simulink model "bebop_full"  (R2019b)
settings: Solver=VariableStepAuto  StartTime=0.0  StopTime=10.0  RelTol=1e-3
values from neighbouring files (symbols this model uses):
  Body_pos_damper = [ld; bd; 0] .* [1, -1, -1, 1;                                   1, 1, -1, -1;                                   0,0,0,0]    [MatToSimulink_test_tutorial.m]
  Damping_matrix_damper = eye(3) .* 1    [MatToSimulink_test_tutorial.m]
  delta_l0_body_frame = [ld; bd; delta_h_damper] .* [1,-1,-1, 1;                                                    1, 1,-1,-1 ... (first row only)    [MatToSimulink_test_tutorial.m]
  Elastic_matrix_damper = eye(3) .* 100    [MatToSimulink_test_tutorial.m]
  g = 9.81    [MatToSimulink_test_tutorial.m]
  Ib = diag([Ixxb, Iyyb, Izzb])    [MatToSimulink_test_tutorial.m]
  iIb = Ib \ eye(3)    [MatToSimulink_test_tutorial.m]
  k_t = 0.01    [MatToSimulink_test_tutorial.m]
  M_c = [b*k_t; l*k_t; k_tau] .* [-1 1 1 -1; 1 1 -1 -1; 1 -1 1 -1]    [MatToSimulink_test_tutorial.m]
  mb = 0.3    [MatToSimulink_test_tutorial.m]
  mc = 0.2    [MatToSimulink_test_tutorial.m]
  omega_c_propeller = 50    [MatToSimulink_test_tutorial.m]
libraries: vrlib x2
settings Model: Creator=ASUS  LastModifiedBy=ASUS

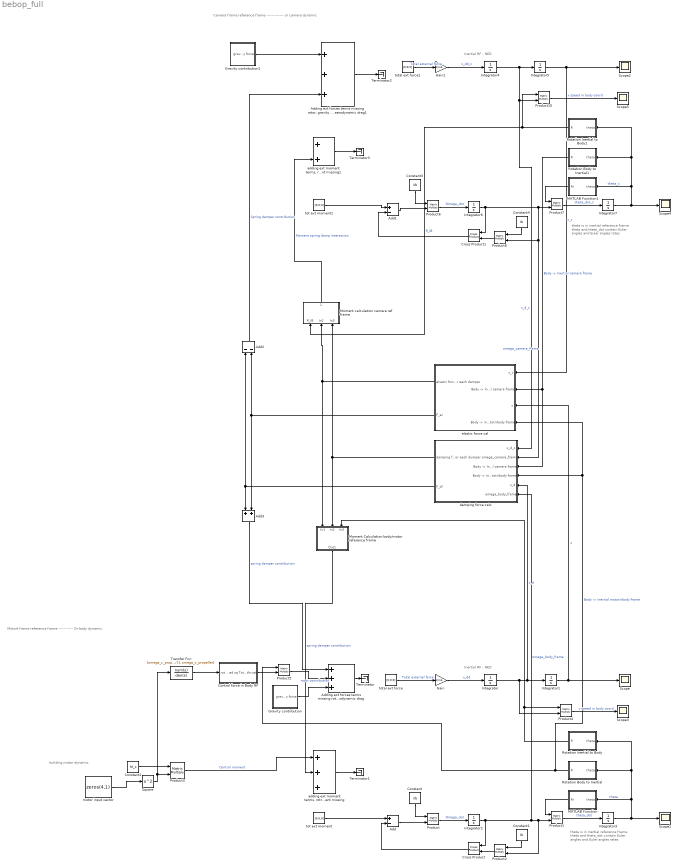
== system bebop_full ==
  note: Motort frame reference frame ----------- Or body dynamic
  note: building motor dynamic
  note: Inertial RF - NED
  note: theta is in inertial
      | reference frame
      |
      | theta and theta_dot contain
      | Euler angles and Euler angles rates
  note: Inertial RF - NED
  note: Camera frame reference frame ------------- or camera dynamic
  note: theta is in inertial
      | reference frame
      |
      | theta and theta_dot contain
      | Euler angles and Euler angles rates
  Add : Sum  Inputs=+-
  Add1 : Sum  Inputs=+-
  Add2 : Sum  Inputs=--
  Add3 : Sum
  "Adding ext forces terms missing rotor, gravity --Inertial Reference frame-- missing aerodynamic drag" : Sum  Inputs=+++
  "Adding ext forces terms missing rotor, gravity --Inertial Reference frame-- missing aerodynamic drag1" : Sum  Inputs=+++
  Constant : Constant  Value=iIb
  Constant1 : Constant  Value=Ib
  Constant2 : Constant  Value=M_c
  Constant3 : Constant  Value=iIb
  Constant4 : Constant  Value=Ib
  Control force in Body RF : Subsystem
  Cross Product : vrlib/Utilities/Cross Product
      settings: SourceProductName=Simulink
  Cross Product1 : vrlib/Utilities/Cross Product
      settings: SourceProductName=Simulink
  Gain : Gain  Gain=1/mb
  Gain1 : Gain  Gain=1/mb
  Gravity contribution : Subsystem
  Gravity contribution1 : Subsystem
  Integrator{,1..7} (8 alike) : Integrator  InitialCondition=[0;0;0]
  MATLAB Function : MATLAB Function  TreatAsAtomicUnit=on
  MATLAB Function1 : MATLAB Function  TreatAsAtomicUnit=on
  Moment Calculation body/motor reference frame : Subsystem
  Moment calculation camera ref frame : Subsystem
  Product{,1..8,10} (10 alike) : Product  Multiplication=Matrix(*)
  Rotation Body to Inertial : MATLAB Function  TreatAsAtomicUnit=on
  Rotation Body to Inertial1 : MATLAB Function  TreatAsAtomicUnit=on
  Rotation Inertial to Body : MATLAB Function  TreatAsAtomicUnit=on
  Rotation Inertial to Body1 : MATLAB Function  TreatAsAtomicUnit=on
  Scope{,1..5} (6 alike) : Scope
  Square : Math  Operator=square  SignedPower=off  SaturateOnIntegerOverflow=on
  Terminator{,1..3} (4 alike) : Terminator
  Transfer Fcn : TransferFcn  Numerator=[omega_c_propeller]  Denominator=[1 omega_c_propeller]
  "adding ext moment terms, rotr precession and aerodynamic moment missing" : Sum  Inputs=+++
  "adding ext moment terms, rotr precession and aerodynamic moment missing1" : Sum
  damping force calc : Subsystem
  elastic force cal : Subsystem
  "motor input vector " : Constant  Value=zeros(4,1)
  tot ext moment : Constant  Value=[0;0;0]
  tot ext moment1 : Constant  Value=[0;0;0]
  total ext force : Constant  Value=[0;0;0]
  total ext force1 : Constant  Value=[0;0;0]
  wires:
  Integrator/1 -> damping force calc/5(x_d), Integrator1/1, Product4/2  "x_d"
  Gain/1 -> Integrator/1  "x_dd"
  Integrator1/1 -> Scope/1, elastic force cal/3(x)  "x"
  total ext force/1 -> Gain/1  "Total external force"
  Product/1 -> Integrator2/1  "Omega_dot"
  tot ext moment/1 -> Add/1
  Constant/1 -> Product/1
  Add/1 -> Product/2
  Integrator2/1 -> Cross Product/1, damping force calc/6(omega_body_frame), Product2/2, Product1/2  "omega_body_frame"
  Integrator3/1 -> Rotation Inertial to Body/1(theta), Rotation Body to Inertial/1(theta), MATLAB Function/1(theta), Scope1/1  "theta"
  Product1/1 -> Integrator3/1  "theta_dot"
  MATLAB Function/1(Rr) -> Product1/1
  Product2/1 -> Cross Product/2
  Cross Product/1 -> Add/2
  Constant1/1 -> Product2/1
  Rotation Inertial to Body/1(R) -> Moment Calculation body/motor reference frame/3(In3), Product4/1
  Product4/1 -> Scope3/1  "v speed in body coord"
  Rotation Body to Inertial/1(R) -> elastic force cal/4("Body -> inertial mototr/body frame"), damping force calc/4("Body -> inertial mototr/body frame"), Product5/1  "Body -> inertial mototr/body frame"
  "motor input vector "/1 -> Square/1
  Constant2/1 -> Product3/1
  Product3/1 -> "adding ext moment terms, rotr precession and aerodynamic moment missing"/1  "Control moment"
  "adding ext moment terms, rotr precession and aerodynamic moment missing"/1 -> Terminator1/1
  Square/1 -> Transfer Fcn/1, Product3/2
  Product5/1 -> "Adding ext forces terms missing rotor, gravity --Inertial Reference frame-- missing aerodynamic drag"/2  "rotot contribution"
  Gravity contribution/1("gravity force ") -> "Adding ext forces terms missing rotor, gravity --Inertial Reference frame-- missing aerodynamic drag"/3
  "Adding ext forces terms missing rotor, gravity --Inertial Reference frame-- missing aerodynamic drag"/1 -> Terminator/1
  Control force in Body RF/1(Total thrust) -> Product5/2
  Add1/1 -> Product6/2
  Cross Product1/1 -> Add1/2
  "adding ext moment terms, rotr precession and aerodynamic moment missing1"/1 -> Terminator3/1
  Constant3/1 -> Product6/1
  Product7/1 -> Integrator7/1  "theta_dot_c"
  Rotation Inertial to Body1/1(R) -> Moment calculation camera ref frame/1(R_IB), Product10/1  "R_IB"
  Gravity contribution1/1("gravity force ") -> "Adding ext forces terms missing rotor, gravity --Inertial Reference frame-- missing aerodynamic drag1"/1
  Product8/1 -> Cross Product1/2
  MATLAB Function1/1(Rr) -> Product7/1
  tot ext moment1/1 -> Add1/1
  Product10/1 -> Scope5/1  "v speed in body coord"
  Integrator5/1 -> elastic force cal/1(x_c), Scope2/1  "x_c"
  Integrator6/1 -> Cross Product1/1, damping force calc/2(omega_camera_frame), Product8/2, Product7/2  "omega_camera_frame"
  Integrator7/1 -> Rotation Inertial to Body1/1(theta), Rotation Body to Inertial1/1(theta), MATLAB Function1/1(theta), Scope4/1  "theta_c"
  total ext force1/1 -> Gain1/1  "Total external force"
  Constant4/1 -> Product8/1
  Product6/1 -> Integrator6/1  "Omega_dot"
  "Adding ext forces terms missing rotor, gravity --Inertial Reference frame-- missing aerodynamic drag1"/1 -> Terminator2/1
  Gain1/1 -> Integrator4/1  "x_dd_c"
  Integrator4/1 -> damping force calc/1(x_d_c), Product10/2, Integrator5/1  "x_d_c"
  Rotation Body to Inertial1/1(R) -> damping force calc/3("Body -> Inertial camera frame"), elastic force cal/2("Body -> Inertial camera frame")  "Body -> Inertial camera frame"
  elastic force cal/1(elsatic force components for each damper) -> Moment calculation camera ref frame/2(In2), Moment Calculation body/motor reference frame/1(In1)
  elastic force cal/2(F_eI) -> Add2/2, Add3/2
  damping force calc/1(damping force components for each dumper) -> Moment Calculation body/motor reference frame/2(In2), Moment calculation camera ref frame/3(In3)
  damping force calc/2(F_dI) -> Add3/1, Add2/1
  Add2/1 -> "Adding ext forces terms missing rotor, gravity --Inertial Reference frame-- missing aerodynamic drag1"/3  "Spring damper contribution"
  Add3/1 -> "Adding ext forces terms missing rotor, gravity --Inertial Reference frame-- missing aerodynamic drag"/1  "spring damper contribution"
  Moment calculation camera ref frame/1(Spring-damper moment contribution) -> "adding ext moment terms, rotr precession and aerodynamic moment missing1"/2  "Moment spring damp interaction"
  Moment Calculation body/motor reference frame/1(Out1) -> "adding ext moment terms, rotr precession and aerodynamic moment missing"/2  "spring damper contribution"
  Transfer Fcn/1 -> Control force in Body RF/1(rot speed sq)

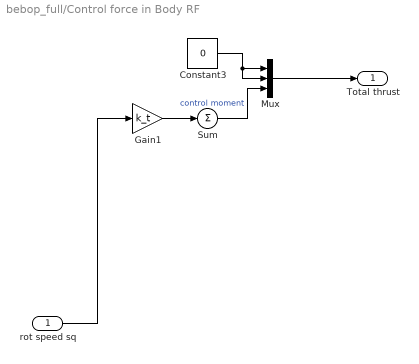
== system bebop_full/Control force in Body RF ==
  rot speed sq : Inport
  Constant3 : Constant  Value=0
  Gain1 : Gain  Gain=k_t
  Mux : Mux  Inputs=3
  Sum : Sum  Inputs=+
  Total thrust : Outport
  wires:
  Sum/1 -> Mux/3  "control moment"
  Constant3/1 -> Mux/1, Mux/2
  Mux/1 -> Total thrust/1
  Gain1/1 -> Sum/1
  rot speed sq/1 -> Gain1/1

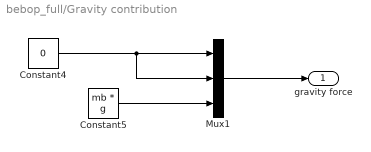
== system bebop_full/Gravity contribution ==
  Constant4 : Constant  Value=0
  Constant5 : Constant  Value=mb * g
  Mux1 : Mux  Inputs=3
  "gravity force " : Outport
  wires:
  Constant4/1 -> Mux1/1, Mux1/2
  Constant5/1 -> Mux1/3
  Mux1/1 -> "gravity force "/1

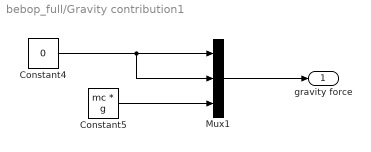
== system bebop_full/Gravity contribution1 ==
  Constant4 : Constant  Value=0
  Constant5 : Constant  Value=mc * g
  Mux1 : Mux  Inputs=3
  "gravity force " : Outport
  wires:
  Constant4/1 -> Mux1/1, Mux1/2
  Constant5/1 -> Mux1/3
  Mux1/1 -> "gravity force "/1

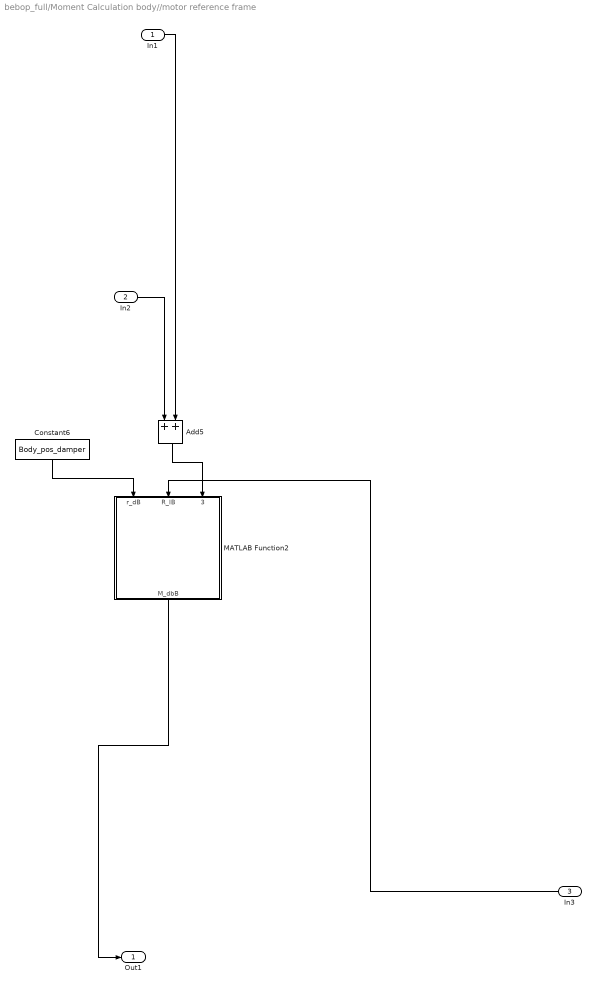
== system bebop_full/Moment Calculation body//motor reference frame ==
  In1 : Inport
  In2 : Inport  Port=2
  In3 : Inport  Port=3
  Add5 : Sum
  Constant6 : Constant  Value=Body_pos_damper
  MATLAB Function2 : MATLAB Function  TreatAsAtomicUnit=on
  Out1 : Outport
  wires:
  Add5/1 -> MATLAB Function2/3(F_dbI_comp)
  In1/1 -> Add5/2
  In2/1 -> Add5/1
  In3/1 -> MATLAB Function2/2(R_IB)
  Constant6/1 -> MATLAB Function2/1(r_dB)
  MATLAB Function2/1(M_dbB) -> Out1/1

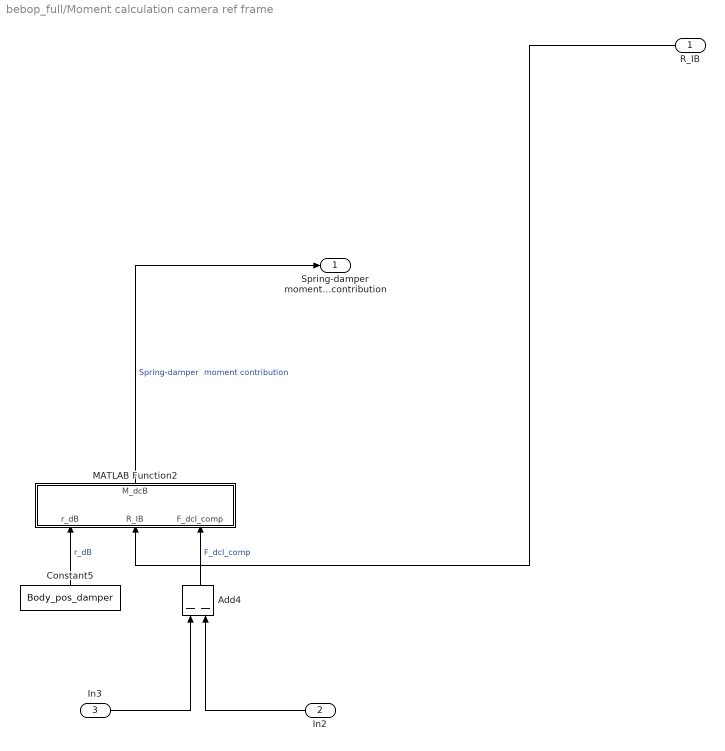
== system bebop_full/Moment calculation camera ref frame ==
  R_IB : Inport
  In2 : Inport  Port=2
  In3 : Inport  Port=3
  Add4 : Sum  Inputs=--
  Constant5 : Constant  Value=Body_pos_damper
  MATLAB Function2 : MATLAB Function  TreatAsAtomicUnit=on
  Spring-damper moment contribution : Outport
  wires:
  Add4/1 -> MATLAB Function2/3(F_dcI_comp)  "F_dcI_comp"
  MATLAB Function2/1(M_dcB) -> Spring-damper moment contribution/1  "Spring-damper  moment contribution"
  In3/1 -> Add4/1
  Constant5/1 -> MATLAB Function2/1(r_dB)  "r_dB"
  R_IB/1 -> MATLAB Function2/2(R_IB)
  In2/1 -> Add4/2

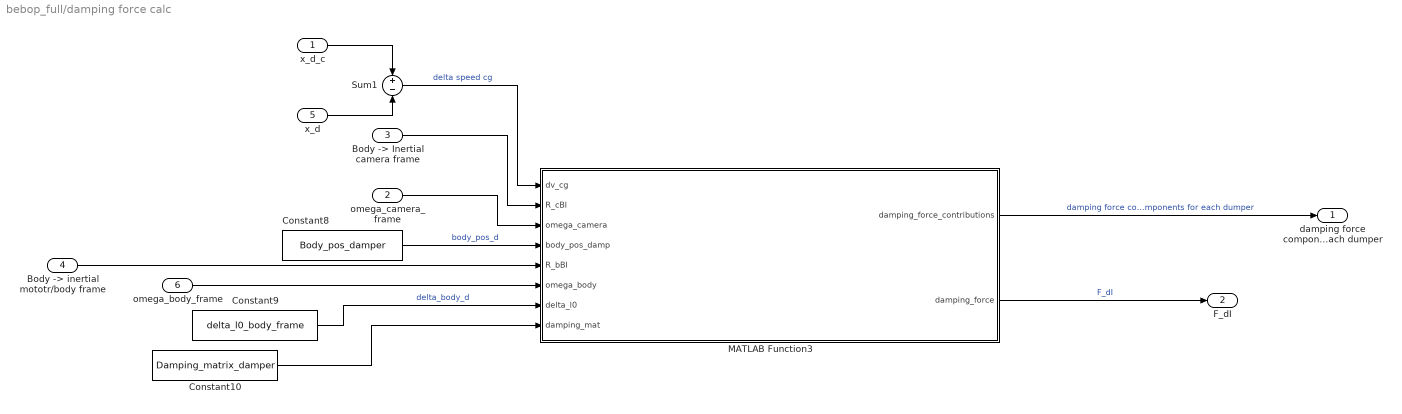
== system bebop_full/damping force calc ==
  x_d_c : Inport
  omega_camera_frame : Inport  Port=2
  "Body -> Inertial camera frame" : Inport  Port=3
  "Body -> inertial mototr/body frame" : Inport  Port=4
  x_d : Inport  Port=5
  omega_body_frame : Inport  Port=6
  Constant10 : Constant  Value=Damping_matrix_damper
  Constant8 : Constant  Value=Body_pos_damper
  Constant9 : Constant  Value=delta_l0_body_frame
  MATLAB Function3 : MATLAB Function  TreatAsAtomicUnit=on
  Sum1 : Sum  Inputs=+-
  damping force components for each dumper : Outport
  F_dI : Outport  Port=2
  wires:
  MATLAB Function3/2(damping_force) -> F_dI/1  "F_dI"
  x_d/1 -> Sum1/2
  x_d_c/1 -> Sum1/1
  "Body -> inertial mototr/body frame"/1 -> MATLAB Function3/5(R_bBI)
  omega_body_frame/1 -> MATLAB Function3/6(omega_body)
  omega_camera_frame/1 -> MATLAB Function3/3(omega_camera)
  Constant8/1 -> MATLAB Function3/4(body_pos_damp)  "body_pos_d"
  MATLAB Function3/1(damping_force_contributions) -> damping force components for each dumper/1  "damping force components for each dumper"
  Sum1/1 -> MATLAB Function3/1(dv_cg)  "delta speed cg"
  Constant10/1 -> MATLAB Function3/8(damping_mat)
  "Body -> Inertial camera frame"/1 -> MATLAB Function3/2(R_cBI)
  Constant9/1 -> MATLAB Function3/7(delta_l0)  "delta_body_d"

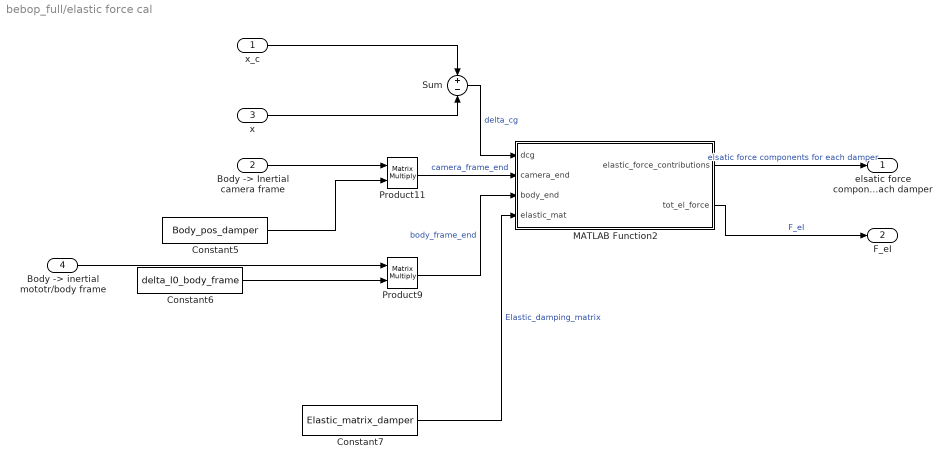
== system bebop_full/elastic force cal ==
  x_c : Inport
  "Body -> Inertial camera frame" : Inport  Port=2
  x : Inport  Port=3
  "Body -> inertial mototr/body frame" : Inport  Port=4
  Constant5 : Constant  Value=Body_pos_damper
  Constant6 : Constant  Value=delta_l0_body_frame
  Constant7 : Constant  Value=Elastic_matrix_damper
  MATLAB Function2 : MATLAB Function  TreatAsAtomicUnit=on
  Product11 : Product  Multiplication=Matrix(*)
  Product9 : Product  Multiplication=Matrix(*)
  Sum : Sum  Inputs=+-
  elsatic force components for each damper : Outport
  F_eI : Outport  Port=2
  wires:
  Constant6/1 -> Product9/2
  MATLAB Function2/2(tot_el_force) -> F_eI/1  "F_eI"
  "Body -> inertial mototr/body frame"/1 -> Product9/1
  Constant7/1 -> MATLAB Function2/4(elastic_mat)  "Elastic_damping_matrix"
  x_c/1 -> Sum/1
  x/1 -> Sum/2
  MATLAB Function2/1(elastic_force_contributions) -> elsatic force components for each damper/1  "elsatic force components for each damper"
  Product9/1 -> MATLAB Function2/3(body_end)  "body_frame_end"
  Product11/1 -> MATLAB Function2/2(camera_end)  "camera_frame_end"
  Constant5/1 -> Product11/2
  "Body -> Inertial camera frame"/1 -> Product11/1
  Sum/1 -> MATLAB Function2/1(dcg)  "delta_cg"

== matlab function bebop_full/Rotation Inertial to Body ==
  data: theta input; R output
function R = R_ItB(theta)

sp = sin(theta(1));
cp = cos(theta(1));

st = sin(theta(2));
ct = cos(theta(2));

ss = sin(theta(3));
cs = cos(theta(3));

R_Itv1 = [cs, ss, 0;...
          -ss, cs, 0;...
          0, 0, 1];

R_v1tv2 = [ct, 0, -st;...
           0, 1, 0;
           st, 0, ct];
       
R_v2tB = [1, 0, 0;...
          0, cp, sp;...
          0, -sp, cp];
      
R = R_v2tB * R_v1tv2 * R_Itv1;

== matlab function bebop_full/MATLAB Function ==
  data: theta input; Rr output
function Rr = rates_rot_mat(theta)

Rr = [1, sin(theta(1)).*tan(theta(2)), cos(theta(1)).*tan(theta(2));...
      0, cos(theta(1)), -sin(theta(1));...
      0, sin(theta(1))./cos(theta(2)), cos(theta(1))./cos(theta(2)) ];

== matlab function bebop_full/Rotation Body to Inertial ==
  data: theta input; R output
function R = R_BtI(theta)

sp = sin(-theta(1));
cp = cos(-theta(1));

st = sin(-theta(2));
ct = cos(-theta(2));

ss = sin(-theta(3));
cs = cos(-theta(3));

R_Itv1 = [cs, ss, 0;...
          -ss, cs, 0;...
          0, 0, 1];

R_v1tv2 = [ct, 0, -st;...
           0, 1, 0;
           st, 0, ct];
       
R_v2tB = [1, 0, 0;...
          0, cp, sp;...
          0, -sp, cp];
      
R =  R_Itv1 * R_v1tv2 * R_v2tB;

== matlab function bebop_full/MATLAB Function1 ==
  data: theta input; Rr output
function Rr = rates_rot_mat(theta)

Rr = [1, sin(theta(1)).*tan(theta(2)), cos(theta(1)).*tan(theta(2));...
      0, cos(theta(1)), -sin(theta(1));...
      0, sin(theta(1))./cos(theta(2)), cos(theta(1))./cos(theta(2)) ];

== matlab function bebop_full/Rotation Body to Inertial1 ==
  data: theta input; R output
function R = R_BtI(theta)

sp = sin(-theta(1));
cp = cos(-theta(1));

st = sin(-theta(2));
ct = cos(-theta(2));

ss = sin(-theta(3));
cs = cos(-theta(3));

R_Itv1 = [cs, ss, 0;...
          -ss, cs, 0;...
          0, 0, 1];

R_v1tv2 = [ct, 0, -st;...
           0, 1, 0;
           st, 0, ct];
       
R_v2tB = [1, 0, 0;...
          0, cp, sp;...
          0, -sp, cp];
      
R =  R_Itv1 * R_v1tv2 * R_v2tB;

== matlab function bebop_full/Rotation Inertial to Body1 ==
  data: theta input; R output
function R = R_ItB(theta)

sp = sin(theta(1));
cp = cos(theta(1));

st = sin(theta(2));
ct = cos(theta(2));

ss = sin(theta(3));
cs = cos(theta(3));

R_Itv1 = [cs, ss, 0;...
          -ss, cs, 0;...
          0, 0, 1];

R_v1tv2 = [ct, 0, -st;...
           0, 1, 0;
           st, 0, ct];
       
R_v2tB = [1, 0, 0;...
          0, cp, sp;...
          0, -sp, cp];
      
R = R_v2tB * R_v1tv2 * R_Itv1;

== matlab function bebop_full/elastic force cal/MATLAB Function2 ==
  data: dcg input; elastic_force_contributions output; camera_end input; body_end input; elastic_mat input; tot_el_force output
function [elastic_force_contributions, tot_el_force]= el_force_contr_calc(dcg, camera_end, body_end, elastic_mat)

elastic_force_contributions = elastic_mat * ([dcg, dcg, dcg, dcg] + camera_end - body_end);

tot_el_force = sum(elastic_force_contributions, 2);

== matlab function bebop_full/damping force calc/MATLAB Function3 ==
  data: dv_cg input; damping_force_contributions output; R_cBI input; omega_camera input; body_pos_damp input; R_bBI input; omega_body input; delta_l0 input; damping_mat input; damping_force output
function [damping_force_contributions, damping_force]= damping_force_calc(dv_cg, R_cBI, omega_camera, body_pos_damp, R_bBI, omega_body, delta_l0, damping_mat)


damping_force_contributions = damping_mat * ([dv_cg, dv_cg, dv_cg, dv_cg,] + R_cBI * skew(omega_camera) * body_pos_damp ...
                                             - R_bBI * skew(omega_body) * delta_l0);

damping_force = sum(damping_force_contributions, 2);

== matlab function bebop_full/Moment calculation camera ref frame/MATLAB Function2 ==
  data: r_dB input; R_IB input; M_dcB output; F_dcI_comp input
function M_dcB = Moment_B(r_dB, R_IB, F_dcI_comp)

M_dcB = sum(cross(r_dB, R_IB * F_dcI_comp),2);

== matlab function bebop_full/Moment Calculation body//motor reference frame/MATLAB Function2 ==
  data: r_dB input; R_IB input; M_dbB output; F_dbI_comp input
function M_dbB = Moment_bB(r_dB, R_IB, F_dbI_comp)

M_dbB = sum(cross(r_dB, R_IB * F_dbI_comp),2);
